simulink subsystem "yarn_alarms"  (R2023b)
settings: Solver=VariableStepAuto  StartTime=0.0  StopTime=10.0  RelTol=1e-3
values from neighbouring files (symbols this model uses):
  d_res = 7    [mdl_parameters_int.mat]
  delta = 0.177250403315    [mdl_parameters_int.mat]
  l_hf = 10.5    [mdl_parameters_int.mat]
  tau_s = 0.0005    [mdl_parameters_int.mat]
settings Model: Creator=Previ  LastModifiedBy=Previ

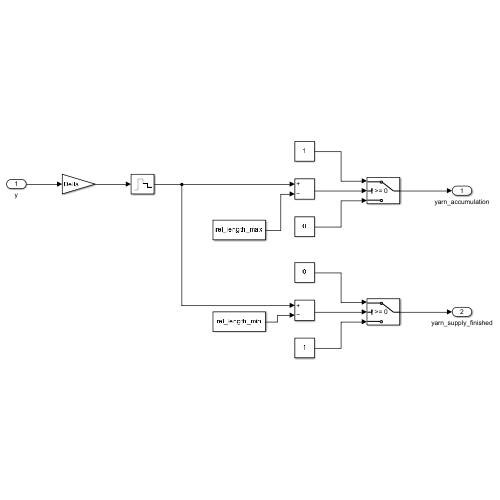
[thumbnail: Simulink's stored preview of the top-level diagram]
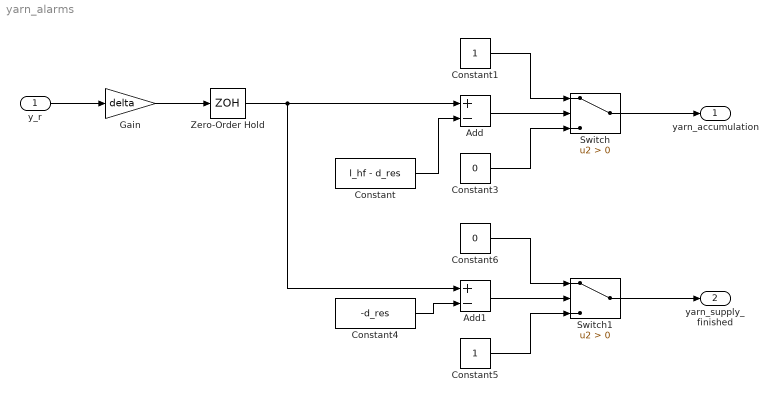
== system yarn_alarms ==
  y_r : Inport  PortDimensions=[1, 1]
  Add : Sum  Inputs=+-
  Add1 : Sum  Inputs=+-
  Constant : Constant  Value=l_hf - d_res
  Constant1 : Constant
  Constant3 : Constant  Value=0
  Constant4 : Constant  Value=-d_res
  Constant5 : Constant
  Constant6 : Constant  Value=0
  Gain : Gain  Gain=delta
  Switch : Switch  Criteria=u2 > Threshold  SaturateOnIntegerOverflow=off  InputSameDT=off
  Switch1 : Switch  Criteria=u2 > Threshold  SaturateOnIntegerOverflow=off  InputSameDT=off
  Zero-Order Hold : ZeroOrderHold  SampleTime=tau_s
  yarn_accumulation : Outport  PortDimensions=[1, 1]
  yarn_supply_finished : Outport  Port=2  PortDimensions=[1, 1]
  wires:
  Constant5/1 -> Switch1/3
  y_r/1 -> Gain/1
  Add1/1 -> Switch1/2
  Constant3/1 -> Switch/3
  Constant1/1 -> Switch/1
  Constant4/1 -> Add1/2
  Zero-Order Hold/1 -> Add1/1, Add/1
  Switch1/1 -> yarn_supply_finished/1
  Switch/1 -> yarn_accumulation/1
  Gain/1 -> Zero-Order Hold/1
  Constant/1 -> Add/2
  Add/1 -> Switch/2
  Constant6/1 -> Switch1/1
